simulink model "FullFMS_2026_02_25_V0_4_11"  (R2026a)
(part 4 of 5)

  data: Control_80 input Bus: B_Control_80; Actuators_80 input Bus: B_Actuators_80; Sensors_80 input Bus: B_Sensors_80; AS_i_70 input Bus: B_AS_i_70; Control_70 input Bus: B_Control_70; Actuators_70 input Bus: B_Actuators_70; Sensors_70 input Bus: B_Sensors_70; C_82_Profibus local; C_83_RQ_Parts local; C_85_Continuous local; C_85_Counted local; C_85_Initialization local; C_85_Part_Del local; C_85_Single local; C_85_Start local; F_82_Arm_2_Del local; F_82_Arm_2_Mag local; F_82_Pist_Adv local; F_82_Suction_Off local; F_82_Suction_On local; F_83_Led_Extra1 local; F_83_Led_Extra2 local; F_83_Led_Reset local; F_83_Led_Start local; F_83_Panel_O4 local; F_83_Panel_O5 local; F_83_Panel_O6 local; F_83_Panel_O7 local; O_80_Arm_Del local; O_80_Arm_Mag local; O_80_Mag_Empty local; O_80_Mag_Full local; O_80_Part_Stuck local; O_80_Pist_Back local; O_80_Pist_Fwd local; O_81_Key_Pos local; O_81_Panel_I4 local; O_81_Panel_I5 local; O_81_Panel_I6 local; O_81_Panel_I7 local; O_81_Reset local; O_81_Start local; O_81_Stop local; C_75_ID_Delivery1 local; C_75_ID_Delivery2 local; C_75_Identified local; C_75_Identified80 local; C_75_Initialization local; C_75_Part_Del local; C_75_RQ_Delivery1 local; C_75_RQ_Delivery2 local; C_75_RQ_Part_Del local; C_75_RQ_Wrong local; C_75_Requested local; C_75_Requested80 local; F_72_Air_On local; F_72_Eject_Part local; F_72_Elev_Down local; F_72_Elev_Up local; F_73_Led_Extra1 local; F_73_Led_Extra2 local; F_73_Led_Reset local; F_73_Led_Start local; F_73_Panel_O4 local; F_73_Panel_O5 local; F_73_Panel_O6 local; F_73_Panel_O7 local; O_70_Elev_High local; O_70_Elev_Low local; O_70_Pist_Back local; O_70_SInductive local; O_70_SPart local; O_70_SPart_Height local; O_70_SStation local; O_71_Key_Pos local; O_71_Panel_I4 local; O_71_Panel_I5 local; O_71_Panel_I6 local; O_71_Panel_I7 local; O_71_Reset local; O_71_Start local; O_71_Stop local; A_73_TestCartID local; A_74_CRoute_In local; A_74_CRoute_In80 local; A_74_CRoute_Out local; A_74_Cart_Full local; A_74_Cart_Next local; A_74_Cart_Stat local; A_74_Count local; A_74_No_Cart local; A_74_Optic local; A_74_Pist_Bck local; A_74_Release_FB local; A_74_Request local; C_72_Profibus local; AS_i_30 input Bus: B_AS_i_30; AS_i_50 input Bus: B_AS_i_50; AS_i_90 input Bus: B_AS_i_90; Actuators_100 input Bus: B_Actuators_100; Actuators_20 input Bus: B_Actuators_20; Actuators_30 input Bus: B_Actuators_30; Actuators_50 input Bus: B_Actuators_50; Actuators_60 input Bus: B_Actuators_60; Actuators_90 input Bus: B_Actuators_90; Control_100 input Bus: B_Control_100; Control_20 input Bus: B_Control_20; Control_30 input Bus: B_Control_30; Control_50 input Bus: B_Control_50; Control_60 input Bus: B_Control_60; Control_90 input Bus: B_Control_90; Sensors_100 input Bus: B_Sensors_100; Sensors_20 input Bus: B_Sensors_20; Sensors_30 input Bus: B_Sensors_30; Sensors_50 input Bus: B_Sensors_50; Sensors_60 input Bus: B_Sensors_60; Sensors_90 input Bus: B_Sensors_90; A_32_RoboCartID local; A_34_CRoute_In local; A_34_CRoute_Out local; A_34_Cart_Full local; A_34_Cart_Next local; A_34_Cart_Stat local; A_34_Count local; A_34_No_Cart local; A_34_Optic local; A_34_Pist_Bck local; A_34_Release_FB local; A_34_Request local; A_53_SortCartID local; A_54_CRoute_In local; A_54_CRoute_Out local; A_54_Cart_Full local; A_54_Cart_Next local; A_54_Cart_Stat local; A_54_Count local; A_54_No_Cart local; A_54_Optic local; A_54_Pist_Bck local; A_54_Release_FB local; A_54_Request local; A_93_ProcCartID local; A_94_CRoute_In local; A_94_CRoute_Out local; A_94_Cart_Full local; A_94_Cart_Next local; A_94_Cart_Stat local; A_94_Count local; A_94_No_Cart local; A_94_Optic local; A_94_Pist_Bck local; A_94_Release_FB local; A_94_Request local; C_102_Profibus local; C_103_RQ_Turns local; C_105_Initialization local; C_105_Part_ready local; C_105_Rotation local; C_105_Start local; C_105_Test local; C_105_TestDrill local; C_105_Test_Fail local; C_105_Test_Ok local; C_24_CRoute_In local; C_24_CRoute_Out local; C_24_CartDel local; C_24_Request local; C_25_CRoute_In local; C_25_CRoute_Out local; C_25_CartDel local; C_25_Request local; C_26_CRoute_In local; C_26_CRoute_Out local; C_26_CartDel local; C_26_Request local; C_27_CRoute_In local; C_27_CRoute_Out local; C_27_CartDel local; C_27_Request local; C_28_CRoute_In local; C_28_CRoute_Out local; C_28_CartDel local; C_28_Request local; C_29_CRoute_In local; C_29_CRoute_Out local; C_29_CartDel local; C_29_Request local; C_30_Robot1 local; C_30_Robot2 local; C_35_Part_Del local; C_52_Profibus local; C_55_Cart2Del local; C_55_Initialization local; C_55_PD_Sort local; C_55_Start local; C_62_Profibus local; C_65_BRS_Output local; C_65_BSR_Output local; C_65_ID_1 local; C_65_ID_2 local; C_65_Initialization local; C_65_RBS_Output local; C_65_RSB_Output local; C_65_SBR_Output local; C_65_SRB_Output local; C_92_Profibus local; C_95_Cart2Del local; C_95_Del2Cart local; C_95_Initialization local; C_95_PD_Cart local; C_95_PD_Proc local; C_95_Start local; F_102_Drill_Down local; F_102_Drill_On local; F_102_Drill_Pin local; F_102_Drill_Up local; F_102_RT_On local; F_102_Test_Pin local; F_103_Led_Extra1 local; F_103_Led_Extra2 local; F_103_Led_Reset local; F_103_Led_Start local; F_103_Panel_O4 local; F_103_Panel_O5 local; F_103_Panel_O6 local; F_103_Panel_O7 local; F_22_Led_Off local; F_22_Led_On local; F_24_Release_FB local; F_25_Release_FB local; F_26_Release_FB local; F_27_Release_FB local; F_28_Release_FB local; F_29_Release_FB local; F_33_Cover_Cyl local; F_33_Led_Extra1 local; F_33_Led_Extra2 local; F_33_Led_Reset local; F_33_Led_Start local; F_33_Spring_Cyl local; F_52_Claw_2_Cart local; F_52_Claw_2_Del local; F_52_Claw_Down local; F_52_Close_Claw local; F_53_Led_Extra1 local; F_53_Led_Extra2 local; F_53_Led_Reset local; F_53_Led_Start local; F_53_Panel_O4 local; F_53_Panel_O5 local; F_53_Panel_O6 local; F_53_Panel_O7 local; F_62_Conveyor local; F_62_Identify local; F_62_P1 local; F_62_P2 local; F_63_Led_Extra1 local; F_63_Led_Extra2 local; F_63_Led_Reset local; F_63_Led_Start local; F_63_Panel_O4 local; F_63_Panel_O5 local; F_63_Panel_O6 local; F_63_Panel_O7 local; F_92_Claw_2_Cart local; F_92_Claw_2_Del local; F_92_Claw_Down local; F_92_Close_Claw local; F_93_Led_Extra1 local; F_93_Led_Extra2 local; F_93_Led_Reset local; F_93_Led_Start local; F_93_Panel_O4 local; F_93_Panel_O5 local; F_93_Panel_O6 local; F_93_Panel_O7 local; O_100_PDrill_Pos local; O_100_PInit_Pos local; O_100_PTest_Ok local; O_100_PTest_Pos local; O_100_RT_Sensor local; O_100_SDrill_High local; O_100_SDrill_Low local; O_101_Key_Pos local; O_101_Panel_I4 local; O_101_Panel_I5 local; O_101_Panel_I6 local; O_101_Panel_I7 local; O_101_Reset local; O_101_Start local; O_101_Stop local; O_20_Controler_On local; O_20_Off local; O_20_On local; O_24_Cart_Next local; O_24_Cart_Stat local; O_24_Count local; O_24_Optic local; O_24_Pist_Bck local; O_25_Cart_Next local; O_25_Cart_Stat local; O_25_Count local; O_25_Optic local; O_25_Pist_Back local; O_26_Cart_Next local; O_26_Cart_Stat local; O_26_Count local; O_26_Optic local; O_26_Pist_Back local; O_27_Cart_Next local; O_27_Cart_Stat local; O_27_Count local; O_27_Optic local; O_27_Pist_Back local; O_28_Cart_Next local; O_28_Cart_Stat local; O_28_Count local; O_28_Optic local; O_28_Pist_Back local; O_29_Cart_Next local; O_29_Cart_Stat local; O_29_Count local; O_29_Optic local; O_29_Pist_Back local; O_31_Orientation local; O_31_Part_in_Claw local; O_31_Reset local; O_31_Start local; O_31_Stop local; O_32_CoMag_Empty local; O_32_Co_Cyl_Bck local; O_32_Co_Cyl_Fwd local; O_32_Co_PickUp local; O_32_Sp_Cyl_Bck local; O_32_Sp_Cyl_Fwd local; O_32_Sp_PickUp local; O_50_Claw_Cart local; O_50_Claw_Del local; O_50_Claw_High local; O_50_Claw_Low local; O_50_Claw_Reserve local; O_50_Part_Reserve local; O_50_Part_in_Claw local; O_51_Key_Pos local; O_51_Panel_I4 local; O_51_Panel_I5 local; O_51_Panel_I6 local; O_51_Panel_I7 local; O_51_Reset local; O_51_Start local; O_51_Stop local; O_60_Part_Pass local; O_60_SL1_Bck local; O_60_SL1_Fwd local; O_60_SL2_Bck local; O_60_SL2_Fwd local; O_60_SPart local; O_60_SPhoto local; O_60_Slnd local; O_61_Key_Pos local; O_61_Panel_I4 local; O_61_Panel_I5 local; O_61_Panel_I6 local; O_61_Panel_I7 local; O_61_Reset local; O_61_Start local; O_61_Stop local; O_90_Claw_Cart local; O_90_Claw_Del local; O_90_Claw_High local; O_90_Claw_Low local; O_90_Claw_Reserve local; O_90_Part_Reserve local; O_90_Part_in_Claw local; O_91_Key_Pos local; O_91_Panel_I4 local; O_91_Panel_I5 local; O_91_Panel_I6 local; O_91_Panel_I7 local; O_91_Reset local; O_91_Start local; O_91_Stop local; F_22_Conveyor local; status6 local; status local; status2 local; status3 local; status4 local; status5 local; status7 local; status1 local; status10 local; status11 local; status12 local; status13 local; status9 local; status8 local; status14 local; LoopDistCont local; Control_40 input Bus: B_Control_40; AS_i_40 input Bus: B_AS_i_40; Actuators_40 input Bus: B_Actuators_40; Sensors_40 input Bus: B_Sensors_40; A_44_CRoute_In local; A_44_CRoute_Out local; A_44_Cart_Full local; A_44_Cart_Next local; A_44_Cart_Stat local; A_44_Count local; A_44_No_Cart local; A_44_Optic local; A_44_Pist_Bck local; A_44_Release_FB local; A_44_Request local; C_42_Profibus local; C_45_Initialization local; C_45_RetrievePart local; C_45_Start local; C_45_StorePart local; F_43_Led_Extra1 local; F_43_Led_Extra2 local; F_43_Led_Reset local; F_43_Led_Start local; F_43_Panel_O4 local; F_43_Panel_O5 local; F_43_Panel_O6 local; F_43_Panel_O7 local; O_41_Key_Pos local; O_41_Panel_I4 local; O_41_Panel_I5 local; O_41_Panel_I6 local; O_41_Panel_I7 local; O_41_Reset local; O_41_Start local; O_41_Stop local; C_86_Mag_Parts local; A_43_StorCartID local; C_85_Part_Mag local; C_87_RQ_MParts local; MetalicPart local; Part_Equal local; Part_Different local; status15 local; status16 local; status18 local; status17 local; status19 local; S1_3 local; S1_2 local; S1_1 local; S1_5 local; S1_6 local; S1_4 local; Status1_7 local boolean; Status1_4 local boolean; Status1_2 local boolean; Status1_3 local boolean; Status1_6 local boolean; Status1_5 local boolean; Status1_1 local boolean; Status3a_14 local boolean; Status3a_9 local boolean; Status3a_15 local boolean; Status3b_14 local boolean; Status3b_9 local boolean; Status3b_20 local boolean; Status3b_13 local boolean; Status3b_1 local boolean; Status3b15 local boolean; Status3b_15 local boolean; Status3a_4 local boolean; Status3a_6 local boolean; Status3a_5 local boolean; Status3a_10 local boolean; Status3a_12 local boolean; Status3a_11 local boolean; Status3a_7 local boolean; Status3a_3 local boolean; Status3a_2 local boolean; Status3b_7 local boolean; Status3b_5 local boolean; Status3b_6 local boolean; Status3b_18 local boolean; Status3b_19 local boolean; Status3b_12 local boolean; Status3b_11 local boolean; Status3b_10 local boolean; Status3b_2 local boolean; Status3b_3 local boolean; Status3b_4 local boolean; Status3b_8 local boolean; Status3b_17 local boolean; Status3b_16 local boolean; StatusRBS_1 local boolean; StatusRBS_2 local boolean; StatusRBS_3 local boolean; StatusRBS_4 local boolean; StatusRBS_5 local boolean; StatusRSB_1 local boolean; StatusRSB_2 local boolean; StatusRSB_3 local boolean; StatusRSB_4 local boolean; StatusRSB_5 local boolean; StatusBRS_1 local boolean; StatusBRS_2 local boolean; StatusBRS_3 local boolean; StatusBRS_4 local boolean; StatusBRS_5 local boolean; StatusBSR_1 local boolean; StatusBSR_2 local boolean; StatusBSR_3 local boolean; StatusBSR_4 local boolean; StatusBSR_5 local boolean; StatusSRB_1 local boolean; StatusSRB_2 local boolean; StatusSRB_3 local boolean; StatusSRB_4 local boolean; StatusSRB_5 local boolean; StatusSBR_1 local boolean; StatusSBR_2 local boolean; StatusSBR_3 local boolean; StatusSBR_4 local boolean; StatusSBR_5 local boolean; St_C2P0_4_1 local boolean; St_C2P0_4_2 local boolean; St_C2P0_4_3 local boolean; St_C2P0_4_4 local boolean; St_C2P0_4_5 local boolean; St_C2P0_4_6 local boolean; St_C2P0_4_7 local boolean; St_C2P0_4_8 local boolean; St_C2P0_4_9 local boolean; St_C2P1_4_1 local boolean; St_C2P1_4_2 local boolean; St_C2P1_4_3 local boolean; St_C2P1_4_4 local boolean; St_C2P1_4_5 local boolean; St_C2P1_4_6 local boolean; St_C2P1_4_7 local boolean; St_C2P1_4_8 local boolean; St_C2P1_4_9 local boolean; St_C2P2_4_1 local boolean; St_C2P2_4_2 local boolean; St_C2P2_4_3 local boolean; St_C2P2_4_4 local boolean; St_C2P2_4_5 local boolean; St_C2P2_4_6 local boolean; St_C2P2_4_7 local boolean; St_C2P2_4_8 local boolean; St_C2P2_4_9 local boolean; St_C2P3_4_1 local boolean; St_C2P3_4_2 local boolean; St_C2P3_4_3 local boolean; St_C2P3_4_4 local boolean; St_C2P3_4_5 local boolean; St_C2P3_4_6 local boolean; St_C2P3_4_7 local boolean; St_C2P3_4_8 local boolean; St_C2P3_4_9 local boolean; St_C2P4_4_1 local boolean; St_C2P4_4_2 local boolean; St_C2P4_4_3 local boolean; St_C2P4_4_4 local boolean; St_C2P4_4_5 local boolean; St_C2P4_4_6 local boolean; St_C2P4_4_7 local boolean; St_C2P4_4_8 local boolean; St_C2P4_4_9 local boolean; St_DCd0_2b_4 local boolean; St_DCd0_2c_1 local boolean; St_DCd0_2c_10 local boolean; St_DCd0_2c_11 local boolean; St_DCd0_2c_12 local boolean; St_DCd0_2c_13 local boolean; St_DCd0_2c_14 local boolean; St_DCd0_2c_15 local boolean; St_DCd0_2c_16 local boolean; St_DCd0_2c_2 local boolean; St_DCd0_2c_3 local boolean; St_DCd0_2c_5 local boolean; St_DCd0_2c_6 local boolean; St_DCd0_2c_7 local boolean; St_DCd0_2c_8 local boolean; St_DCd0_2c_9 local boolean; St_DCt0_2a_1 local boolean; St_DCt0_2b_1 local boolean; St_DCt0_2b_10 local boolean; St_DCt0_2b_11 local boolean; St_DCt0_2b_12 local boolean; St_DCt0_2b_13 local boolean; St_DCt0_2b_14 local boolean; St_DCt0_2b_15 local boolean; St_DCt0_2b_16 local boolean; St_DCt0_2b_2 local boolean; St_DCt0_2b_3 local boolean; St_DCt0_2b_4 local boolean; St_DCt0_2b_5 local boolean; St_DCt0_2b_6 local boolean; St_DCt0_2b_7 local boolean; St_DCt0_2b_8 local boolean; St_DCt0_2b_9 local boolean; St_DSg0_2a_1 local boolean; St_DSg0_2a_10 local boolean; St_DSg0_2a_11 local boolean; St_DSg0_2a_12 local boolean; St_DSg0_2a_13 local boolean; St_DSg0_2a_14 local boolean; St_DSg0_2a_15 local boolean; St_DSg0_2a_16 local boolean; St_DSg0_2a_2 local boolean; St_DSg0_2a_3 local boolean; St_DSg0_2a_4 local boolean; St_DSg0_2a_5 local boolean; St_DSg0_2a_6 local boolean; St_DSg0_2a_7 local boolean; St_DSg0_2a_8 local boolean; St_DSg0_2a_9 local boolean; St_IdDl_3a_1 local boolean; St_IdDl_3a_13 local boolean; St_IdDl_3a_8 local boolean; St_P2P0_5_1 local boolean; St_P2P0_5_10 local boolean; St_P2P0_5_11 local boolean; St_P2P0_5_12 local boolean; St_P2P0_5_13 local boolean; St_P2P0_5_2 local boolean; St_P2P0_5_3 local boolean; St_P2P0_5_4 local boolean; St_P2P0_5_5 local boolean; St_P2P0_5_6 local boolean; St_P2P0_5_7 local boolean; St_P2P0_5_8 local boolean; St_P2P0_5_9 local boolean; St_P2P1_5_1 local boolean; St_P2P1_5_10 local boolean; St_P2P1_5_11 local boolean; St_P2P1_5_12 local boolean; St_P2P1_5_13 local boolean; St_P2P1_5_2 local boolean; St_P2P1_5_3 local boolean; St_P2P1_5_4 local boolean; St_P2P1_5_5 local boolean; St_P2P1_5_6 local boolean; St_P2P1_5_7 local boolean; St_P2P1_5_8 local boolean; St_P2P1_5_9 local boolean; St_Rbt1_5_1 local boolean; St_Rbt1_5_13 local boolean; St_Rbt2_5_1 local boolean; St_Rbt2_5_13 local boolean; St_Retr_5_1 local boolean; St_Retr_5_13 local boolean; St_Stor_5_1 local boolean; St_Stor_5_13 local boolean; St_Visn_5_1 local boolean; St_Visn_5_13 local boolean; St_ROnly_1 local boolean; St_ROnly_2 local boolean; St_ROnly_3 local boolean; St_ROnly_4 local boolean; St_ROnly_5 local boolean; St_TDrill_1 local boolean; St_TDrill_10 local boolean; St_TDrill_11 local boolean; St_TDrill_2 local boolean; St_TDrill_3 local boolean; St_TDrill_4 local boolean; St_TDrill_5 local boolean; St_TDrill_6 local boolean; St_TDrill_7 local boolean; St_TDrill_8 local boolean; St_TDrill_9 local boolean; St_TOnly_1 local boolean; St_TOnly_2 local boolean; St_TOnly_3 local boolean; St_TOnly_4 local boolean; St_TOnly_5 local boolean; St_TOnly_6 local boolean; St_TOnly_7 local boolean; St_H1_1 local boolean; St_H1_2 local boolean; St_H1_3 local boolean; St_H1_4 local boolean; St_H1_5 local boolean; St_H1_6 local boolean; St_H1_7 local boolean; St_H1_8 local boolean; St_H1_9 local boolean
